simulink model "SPWMInv"  (R2016b)
settings: Solver=VariableStepAuto  StartTime=0.0  StopTime=0.1  RelTol=1e-3
libraries: powerlib x28, powerlib_meascontrol x4
settings Model: Creator=Administrator  LastModifiedBy=Administrator

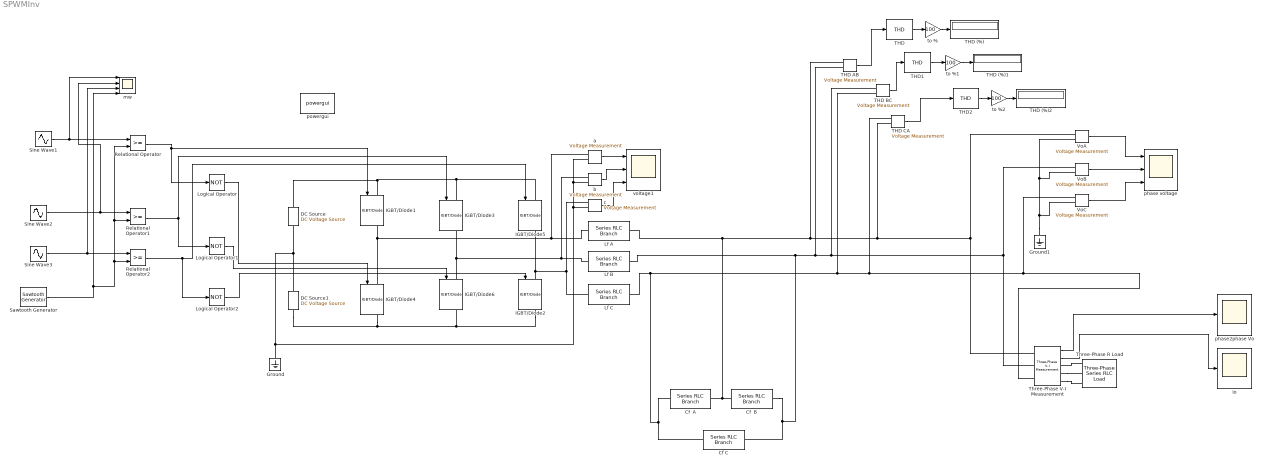
== system SPWMInv ==
  Cf  A : powerlib/Elements/Series RLC Branch  LConnTagsString=__new0  RConnTagsString=__new0  BranchType=C  Resistance=1  Inductance=1e-3  SetiL0=off  InitialCurrent=0  Capacitance=3.82e-7  Setx0=off  InitialVoltage=0  Measurements=None
  Cf  B : powerlib/Elements/Series RLC Branch  LConnTagsString=__new0  RConnTagsString=__new0  BranchType=C  Resistance=1  Inductance=1e-3  SetiL0=off  InitialCurrent=0  Capacitance=3.82e-7  Setx0=off  InitialVoltage=0  Measurements=None
  Cf C : powerlib/Elements/Series RLC Branch  LConnTagsString=__new0  RConnTagsString=__new0  BranchType=C  Resistance=1  Inductance=1e-3  SetiL0=off  InitialCurrent=0  Capacitance=3.82e-7  Setx0=off  InitialVoltage=0  Measurements=None
  DC Source : powerlib/Electrical Sources/DC Voltage Source  Amplitude=710  Measurements=None
  DC Source1 : powerlib/Electrical Sources/DC Voltage Source  Amplitude=710  Measurements=None
  Ground : powerlib/Elements/Ground  LConnTagsString=a
  Ground1 : powerlib/Elements/Ground  LConnTagsString=a
  IGBT/Diode{1..6} (6 alike) : powerlib/Power Electronics/IGBT//Diode  Ron=1e-3  Rs=1e5  Cs=inf  Measurements=on
  Io : Scope
  Lf A : powerlib/Elements/Series RLC Branch  LConnTagsString=__new0  RConnTagsString=__new0  BranchType=L  Resistance=1  Inductance=1.5e-2  SetiL0=off  InitialCurrent=0  Capacitance=1e-6  Setx0=off  InitialVoltage=0  Measurements=None
  Lf B : powerlib/Elements/Series RLC Branch  LConnTagsString=__new0  RConnTagsString=__new0  BranchType=L  Resistance=1  Inductance=1.5e-2  SetiL0=off  InitialCurrent=0  Capacitance=1e-6  Setx0=off  InitialVoltage=0  Measurements=None
  Lf C : powerlib/Elements/Series RLC Branch  LConnTagsString=__new0  RConnTagsString=__new0  BranchType=L  Resistance=1  Inductance=1.5e-2  SetiL0=off  InitialCurrent=0  Capacitance=1e-6  Setx0=off  InitialVoltage=0  Measurements=None
  Logical Operator : Logic  Operator=NOT  Inputs=1  AllPortsSameDT=off  OutDataTypeStr=boolean
  Logical Operator1 : Logic  Operator=NOT  Inputs=1  AllPortsSameDT=off  OutDataTypeStr=boolean
  Logical Operator2 : Logic  Operator=NOT  Inputs=1  AllPortsSameDT=off  OutDataTypeStr=boolean
  Relational Operator : RelationalOperator  OutDataTypeStr=boolean  RndMeth=Simplest
  Relational Operator1 : RelationalOperator  OutDataTypeStr=boolean  RndMeth=Simplest
  Relational Operator2 : RelationalOperator  OutDataTypeStr=boolean  RndMeth=Simplest
  Sawtooth Generator : powerlib_meascontrol/Pulse & Signal Generators/Sawtooth Generator  Freq=14e3  Phase=0  Ts=1/100000
  Sine Wave1 : Sin  Amplitude=0.438  Frequency=100*pi  SampleTime=0
  Sine Wave2 : Sin  Amplitude=0.438  Frequency=100*pi  Phase=-pi*2/3  SampleTime=0
  Sine Wave3 : Sin  Amplitude=0.438  Frequency=100*pi  Phase=pi*2/3  SampleTime=0
  THD : powerlib_meascontrol/Measurements/THD  Freq=50  Ts=0
  THD (%) : Display
      settings: Format=bank
  THD (%)1 : Display
      settings: Format=bank
  THD (%)2 : Display
      settings: Format=bank
  THD AB : powerlib/Measurements/Voltage Measurement  PhasorSimulation=off  OutputType=Complex  PSBequivalent=0
  THD BC : powerlib/Measurements/Voltage Measurement  PhasorSimulation=off  OutputType=Complex  PSBequivalent=0
  THD CA : powerlib/Measurements/Voltage Measurement  PhasorSimulation=off  OutputType=Complex  PSBequivalent=0
  THD1 : powerlib_meascontrol/Measurements/THD  Freq=50  Ts=0
  THD2 : powerlib_meascontrol/Measurements/THD  Freq=50  Ts=0
  Three-Phase R Load : powerlib/Elements/Three-Phase Series RLC Load  LConnTagsString=A|B|C  Configuration=Y (floating)  NominalVoltage=381  Vabc=[1e3 1e3 1e3]  Vabcp=[1e3 1e3 1e3]  NominalFrequency=50  UnbalancedPower=off  ActivePower=11e3  InductivePower=0  CapacitivePower=0  Pabc=[10e3 9e3 11e3]  QLabc=[100 90 110]  QCabc=[100 90 110]  Pabcp=[10e3 9e3 11e3]  QLabcp=[100 90 110]  QCabcp=[100 90 110]  Measurements=None  LoadType=constant Z
  Three-Phase V-I Measurement : powerlib/Measurements/Three-Phase V-I Measurement  VoltageMeasurement=phase-to-phase  SetLabelV=off  LabelV=Vabc  Vpu=off  VpuLL=off  CurrentMeasurement=yes  SetLabelI=off  LabelI=Iabc  Ipu=off  Pbase=100e6  Vbase=500e3  OutputType=Complex  PhasorSimulation=off  PSBequivalent=0
  VoA : powerlib/Measurements/Voltage Measurement  PhasorSimulation=off  OutputType=Complex  PSBequivalent=0
  VoB : powerlib/Measurements/Voltage Measurement  PhasorSimulation=off  OutputType=Complex  PSBequivalent=0
  VoC : powerlib/Measurements/Voltage Measurement  PhasorSimulation=off  OutputType=Complex  PSBequivalent=0
  a : powerlib/Measurements/Voltage Measurement  PhasorSimulation=off  OutputType=Complex  PSBequivalent=0
  b : powerlib/Measurements/Voltage Measurement  PhasorSimulation=off  OutputType=Complex  PSBequivalent=0
  c : powerlib/Measurements/Voltage Measurement  PhasorSimulation=off  OutputType=Complex  PSBequivalent=0
  mw : Scope  NumInputPorts=4
  phase voltage : Scope  NumInputPorts=3
  phase2phase Vo : Scope
  powergui : powerlib/powergui  Priority=1  SimulationMode=Continuous  SolverType=Tustin  SampleTime=50e-6  frequency=60  SPID=off  DisableSnubberDevices=off  DisableRonSwitches=off  DisableVfSwitches=off  SwTol=0  DisplayEquations=off  Interpol=off  ExternalGateDelay=off  methode=off  Ts=10  FunctionMessages=off  echomessages=off  HookPort=off  EnableUseOfTLC=off  x0status=blocks  frequencyindice=0  Pbase=100e6  ErrMax=1e-4  Iterations=50  UnitsV=kV  UnitsW=MW  buscounter=0  RestoreLinks=warning  ResistiveCurrentMeasurement=off  Frange=[0:2:500]  Ylog=off  Xlog=on  ShowGrid=off  save=off  variable=ZData  structure=ScopeData2  ZoomFFT=off  StartTime=0.0  cycles=1  DisplayStyle=1  fundamental=50  FreqAxis=off  MaxFrequency=1000  frequencyindicesteady=1  RmsSteady=1  display=off
  to % : Gain  Gain=100
  to %1 : Gain  Gain=100
  to %2 : Gain  Gain=100
  voltage1 : Scope  NumInputPorts=3
  wires:
  Relational Operator/1 -> Logical Operator/1, IGBT/Diode1/1
  Logical Operator/1 -> IGBT/Diode4/1
  Relational Operator1/1 -> Logical Operator1/1, IGBT/Diode3/1
  Logical Operator1/1 -> IGBT/Diode6/1
  Relational Operator2/1 -> Logical Operator2/1, IGBT/Diode5/1
  Logical Operator2/1 -> IGBT/Diode2/1
  Sine Wave1/1 -> Relational Operator/1, mw/1
  Sawtooth Generator/1 -> Relational Operator1/2, Relational Operator/2, Relational Operator2/2, mw/4
  Sine Wave2/1 -> Relational Operator1/1, mw/2
  Sine Wave3/1 -> Relational Operator2/1, mw/3
  THD/1 -> to %/1
  a/1 -> voltage1/1
  b/1 -> voltage1/2
  c/1 -> voltage1/3
  THD AB/1 -> THD/1
  to %/1 -> THD (%)/1
  VoA/1 -> phase voltage/1
  VoB/1 -> phase voltage/2
  VoC/1 -> phase voltage/3
  THD1/1 -> to %1/1
  THD BC/1 -> THD1/1
  to %1/1 -> THD (%)1/1
  THD2/1 -> to %2/1
  THD CA/1 -> THD2/1
  to %2/1 -> THD (%)2/1
  Three-Phase V-I Measurement/2 -> Io/1
  Three-Phase V-I Measurement/1 -> phase2phase Vo/1
  connections:
  IGBT/Diode2/LConn1 -- Lf C/LConn1 -- c/LConn1 -- IGBT/Diode5/RConn1
  IGBT/Diode2/RConn1 -- DC Source1/LConn1 -- IGBT/Diode4/RConn1 -- IGBT/Diode6/RConn1
  IGBT/Diode6/LConn1 -- Lf B/LConn1 -- b/LConn1 -- IGBT/Diode3/RConn1
  IGBT/Diode4/LConn1 -- a/LConn1 -- Lf A/LConn1 -- IGBT/Diode1/RConn1
  IGBT/Diode1/LConn1 -- DC Source/RConn1 -- IGBT/Diode5/LConn1 -- IGBT/Diode3/LConn1
  a/LConn2 -- b/LConn2 -- c/LConn2 -- Ground/LConn1 -- DC Source/LConn1 -- DC Source1/RConn1
  Cf  B/RConn1 -- Cf  A/LConn1 -- THD CA/LConn2 -- Three-Phase V-I Measurement/LConn1 -- VoA/LConn1 -- THD AB/LConn1 -- Lf A/RConn1
  Cf  A/RConn1 -- THD CA/LConn1 -- VoC/LConn1 -- Three-Phase V-I Measurement/LConn3 -- THD BC/LConn2 -- Lf C/RConn1 -- Cf C/RConn1
  Cf  B/LConn1 -- THD BC/LConn1 -- Three-Phase V-I Measurement/LConn2 -- VoB/LConn1 -- THD AB/LConn2 -- Lf B/RConn1 -- Cf C/LConn1
  Ground1/LConn1 -- VoC/LConn2 -- VoB/LConn2 -- VoA/LConn2
  Three-Phase R Load/LConn1 -- Three-Phase V-I Measurement/RConn1
  Three-Phase V-I Measurement/RConn2 -- Three-Phase R Load/LConn2
  Three-Phase V-I Measurement/RConn3 -- Three-Phase R Load/LConn3
